simulink model "CaptureOutputs_rel"  (R2018b)
settings: Solver=ode4  StartTime=0.0  StopTime=SimEndTime  FixedStep=TimeStep  RelTol=1e-3
model workspace (MATLAB code in the model file):
  | CON = Simulink.Parameter;
  | CON.DataType = 'Bus: Bus_CON';
  | CON.Value = Simulink.Bus.createMATLABStruct('Bus_CON');
undefined symbols (not defined in the file): SampleTime, TimeStep
settings Model: ParameterArgumentNames=CON  OrderedModelArguments=off  Creator=Ethan  LastModifiedBy=Ethan
settings ModelReferenceCC: ModelReferenceNumInstancesAllowed=Single

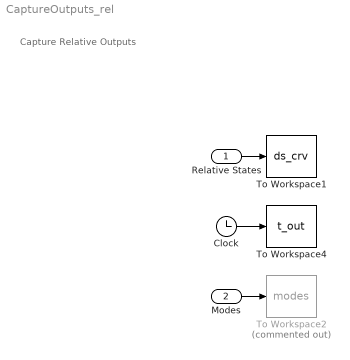
== system CaptureOutputs_rel ==
  note: Capture Relative Outputs
  Relative States : Inport  PortDimensions=6  SampleTime=TimeStep  BusOutputAsStruct=on
  Modes : Inport  Port=2  OutDataTypeStr=Bus: Bus_modes  PortDimensions=1  SampleTime=TimeStep  BusOutputAsStruct=on
  Clock : Clock
  To Workspace1 : ToWorkspace  VariableName=ds_crv  SampleTime=SampleTime
      settings: Save2DSignal=2-D array (concatenate along first dimension)
  To Workspace2 : ToWorkspace  Commented=on  VariableName=modes  SaveFormat=Timeseries  SampleTime=SampleTime
      settings: Save2DSignal=2-D array (concatenate along first dimension)
  To Workspace4 : ToWorkspace  VariableName=t_out  SampleTime=SampleTime
      settings: Save2DSignal=2-D array (concatenate along first dimension)
  wires:
  Relative States/1 -> To Workspace1/1
  Clock/1 -> To Workspace4/1
  Modes/1 -> To Workspace2/1
